simulink model "StateMachinaTesting"  (R2016a)
settings: Solver=VariableStepAuto  StartTime=0.0  StopTime=orbit_length*40  RelTol=1e-3
values from neighbouring files (symbols this model uses):
  A = eye(16,16)    [full_input_list.m]
  B = zeros(16,1)    [full_input_list.m]
  C = blkdiag(eye(3,3),zeros(3,3),eye(10,10))    [full_input_list.m]
  counter = 0    [full_input_list.m]
  deltaT = 0.00001    (= 1e-05)    [full_input_list.m]
  H = C    [full_input_list.m]
  kd = 0.5    [full_input_list.m]    (also in initACS.m = 0.01)
  kp = 1    [full_input_list.m]    (also in initACS.m = 0.01)
  OpModes = [0 0 0]    [full_input_list.m]
  OpTimes = [0 1 2]    [full_input_list.m]
  Q_k = zeros(16,16)    [full_input_list.m]
  R = R_k    [full_input_list.m]
  SeperationTime = 30000    [full_input_list.m]
  sim_start_time = (JD - JD_GPS0) * 24*60*60 - UTC_leap_seconds_wrt_GPS    (= 36000.0287935)    [full_input_list.m]
  st = 1/freq    (= 0.0125)    [full_input_list.m]    (also in initSimulink.m)
  u_k = zeros(16,1)    [full_input_list.m]
  w_k = zeros(16,1)    [full_input_list.m]
  x0 = [0 ... (first row only)    [full_input_list.m]
  Z_k = zeros(16,1)    [full_input_list.m]
undefined symbols (not defined in the file or in its folder): DiscIntNeverNeededParam, Earth, G_igrf, gyro_DCM_BS, H_igrf, I_undeployed, IAU, km, Kschmidt, mag_variance, n, R_mean, sat2, WGS84
libraries: simulink x29, dspmathops x24, aerolibutil x20, aerolibtransform2 x20, vrlib x15, aerolibgravity2 x5, dspinverses x4, SimMainLibrary x3, dspmtrx3 x1, lib_violet_env x1
(part 4 of 4)

== matlab function StateMachinaTesting/Flight Controller/CenterCube EKF/x_measured1/Name change ==
  data: u input; y output
function y = fcn(u)
%#codegen

y = u;

== matlab function StateMachinaTesting/Flight Controller/CenterCube EKF/x_measured1/Name change1 ==
  data: u input; y output
function y = fcn(u)
%#codegen

y = u;

== matlab function StateMachinaTesting/Flight Controller/CenterCube EKF/x_measured1/vis viva ==
  data: x input; xdot output
function xdot = fcn(x)
%#codegen
GM = 3.986e14;
rotation_about_earth = [1;0;0]; % This is assumed for the orbit given by Cory
r = sqrt(x(1)^2+x(2)^2+x(3)^2);
v_mag = sqrt(GM/r);
xdot_cross = cross(rotation_about_earth, x);
xdot_hat = xdot_cross/norm(xdot_cross);
xdot = xdot_hat * v_mag;

== matlab function StateMachinaTesting/x_measured1/Lookup Tables/Sun position off of Jd frm J2000/MATLAB Function ==
  data: J2000_days input; S_ECI output
function S_ECI = sun_position(J2000_days)
% SUN_ECI  Calculate the cartesian coordinates of the sun (in AU)
%			  in the Earth Centered Inertial (ECI) reference frame
%			  with mean equator and equinox of J2000
%
% [S_ECI] = SUN_ECI(J2000_days)
%
% Arguments:
% J2000_days 	- UT Days elapsed since J2000 (1 January, 2000, 12 noon)
% S_ECI				- Sun vector in ECI, units of AU
%
% Todd Humphreys
% Author: Todd Humphreys
% Algorithm: Modified algorithm based on Astronomical Almanac 2001, pg C24
% Tested: Todd Humphreys, November 10, 2001
% 			 Within 0.01 degrees of ECI sun vector from Astronomical Almanac 


RAD = 57.29577951308232;

T   = (J2000_days)/36525;		% Julian centuries since J2000
L0  = (280.46645 + 36000.76983*T + 0.0003032*T^2)/RAD;	% Mean longitude of Sun
M   = (357.52910 + 35999.05030*T - 0.0001559*T^2 - 0.00000048*T^3)/RAD;	 % Mean anomaly
e   = 0.016708617 - 0.000042037*T - 0.0000001236*T^2;
C   = (1.914600 - 0.004817*T - 0.000014*T^2)*sin(M) + (0.019993 - 0.000101*T)*sin(2*M) + 0.000290*sin(3*M);
C   = C/RAD;
SL  = L0 + C;	% Ecliptic longitude
Ni  = M + C;	% Sun true Anomaly
R   = 1.000001018*(1-e^2)/(1+e*cos(Ni));  % Distance, Earth to Sun
SL = SL - (0.01397*T*100)/RAD;	% Correction to ecliptic longitude to reference to J200 equinox
Obl = (23.439291 - 0.0130042*T - 0.00000016*T^2 + 0.000000504*T^3)/RAD;	% Obliquity of ecliptic
SL     = (SL/(2*pi) - floor(SL/(2*pi)))*2*pi;	% Reduce to 2pi range
RA     = atan2(cos(Obl)*sin(SL),cos(SL));		% Right ascension	
Dec    = asin(sin(Obl).*sin(SL));				% Declination

S_ECI = [R*cos(SL); R*cos(Obl)*sin(SL); R*sin(Obl)*sin(SL)];

== matlab function StateMachinaTesting/x_measured1/Name change ==
  data: u input; y output
function y = fcn(u)
%#codegen

y = u;

== matlab function StateMachinaTesting/x_measured1/Name change1 ==
  data: u input; y output
function y = fcn(u)
%#codegen

y = u;

== matlab function StateMachinaTesting/x_measured1/q_N from Sensors/quat From DCM ==
  data: Q input; q_N output; D output
function [q_N,D]  = fcn(Q)

    [V,D] = eig(Q);
    q_N = zeros(4,1);
    a = zeros(3,1);
    tol = 1e-10;
    
    if abs(real(D(1,1))-1) <= tol
        a(:,1) = real(V(:,1));
        phi = atan(abs(imag(D(2,2)))/real(D(2,2)));
    elseif abs(real(D(2,2))-1) <= tol
        a(:,1) = real(V(:,2));
        phi = atan(abs(imag(D(1,1)))/real(D(1,1)));
    elseif abs(real(D(3,3))-1) <= tol
        a(:,1) = real(V(:,3));
        phi = atan(abs(imag(D(1,1)))/real(D(1,1)));
    else 
        a(:,1) = [1;0;0];
        phi = 0;
    end
    
    q_N(1) = a(1)*sin(phi/2);
    q_N(2) = a(2)*sin(phi/2);
    q_N(3) = a(3)*sin(phi/2);
    q_N(4) = cos(phi/2);
end

== matlab function StateMachinaTesting/x_measured1/vis viva ==
  data: x input; xdot output
function xdot = fcn(x)
%#codegen
GM = 3.986e14;
rotation_about_earth = [1;0;0]; % This is assumed for the orbit given by Cory
r = sqrt(x(1)^2+x(2)^2+x(3)^2);
v_mag = sqrt(GM/r);
xdot_cross = cross(rotation_about_earth, x);
xdot_hat = xdot_cross/norm(xdot_cross);
xdot = xdot_hat * v_mag;

== matlab function StateMachinaTesting/MATLAB Function ==
  data: u input; y output
function y = normalizeQuat(u)
%#codegen
y = [u(1:end-4); u(end-3:end)/norm(u(end-3:end))];

== matlab function StateMachinaTesting/SafeMode/ACS State Machine Mode determination ==
  data: SafeMode_In input size=1; SafeMode_Out output; SafedOpMode output; PwbMEX output; t input; ADCSs input; EKFAE input size=13; EKFhs input; OpMode input; PbOpMode input size=1; SeperationCommand input
function [SafeMode_Out, SafedOpMode, PwbMEX] = fcn(SafeMode_In, ...
    t, ADCSs, EKFAE, EKFhs, OpMode, PbOpMode, SeperationCommand)
%#codegen
% x = t, ADCSs, EKFAE, EKFhs, OpMode, PbOpMode, SeperationCommand;
%% States of State Machine
% Time (From Deployment)​           t
% ADCS Health Status​               ADCSs
% EKF Attitude Estimate​            EKFAE
% EKF Health Status​                EKFhs
% Current Status                   OpMode
% PowerBoard Override              PbOpMode
% Deployed or not                  SeperationCommand

%% ADCSs
% ADCS Functional Status            ADCS_Fs
% ADCS Sectional Status             ADCS_Ss
% ADCS Component Status             ADCS_Cs

%%%%%%%%%%%%%%%%%%%%%%%%%%% MODE FLAGS %%%%%%%%%%%%%%%%%%%%%%%%%%%%%%%%%%%%
% 1 = Initial Charging Mode
% 2 = System Verification and Check Mode
% 3 = EPS THS Ping Mode
% 4 = FC THS Ping Mode
% 5 = Detumble Mode
% 6 = Sun Pointing Mode
% 7 = Spin Up Mode
% 8 = End Satellite Deployment Mode
% 9 = Normal OPS Mode
% 10 = Eclipse/Sleep Mode Mode
% 11 = Safe State Mode
% 12 = SeekingEKFConvergence

%% PwbMEX 
% PwbMEX is the error signal sent to the PowerBoard containing important
% information about the status of the ADCSs components as seen in safe
% mode. Informs that Safe Mode was entered, and requests an exit, as well
% as informs of the subsystem components that were not functionoing
% properly.
% MORE INFORMATION TO BE PROVIDED AFTER DISCUSSION WITH PAwwwwwDRAIG ON FORMAT
% AND NEED
SafedOpMode = 0;
SafeMode_Out = 0;
PwbMEX = zeros(1,8);
PwbMEX(1) = 0;
% Contact: Niccolo Porcari 2017

%%%%%%%%%%%%%%%%%%%%%%%%%%%%%%%%%%%%%%%%%%%%%%%%%%%%%%%%%%%%%%%%%%%%%%%%%%
    if t > 2700 % seconds
        % INITIAL CHECKS (check if in SafeMode)
        if (SafeMode_In == true || PbOpMode == 11)
            PwbMEX(1) = 1;
            % FIND A WAY TO INFORM POWERBOARD
            if (PbOpMode ~= 11)
                SafeMode_In = false;
                PwbMEX(1) = 0; % reset error message to powerboard
                OpMode = PbOpMode;
            else
                OpMode = 11;
                %% SAFE MODE OCCURS
                errorPositions = findADCSfault(ADCSs);
                % INFORM POWERBOARD Of location of error
                PwbMEX(2:8) = errorPositions; %%% PARTIAL ONLY
            end
        else
            %% SECTION for all modes where  ADCS is operational 
            % Pretend EKFhs is a boolean for now:
            if (OpMode == 5) || (OpMode == 6) || (OpMode == 7) || (OpMode == 9) || (OpMode == 10)
                if ADCSs(1) == false % Failure of ADCS trips Safe State Mode
                    OpMode = 11;
                    PwbMEX(1) = 1;
                    SafeMode_in = true;
                elseif EKFhs ~= true % Check validity of EKF estimate
                    OpMode = 12;  % Need to think of what we're gonna do if 
                                    % the EKF isn't technically accurate yet
                elseif EKFhs == true
                    OpMode = PbOpMode;
                end
            end
        end
        
        %% RESET OpMode to match PbOpMode 
        if (PbOpMode ~= OpMode && OpMode ~= 12) % set mode to match powerboard demand
            OpMode = PbOpMode;
        end
    end
end
